simulink model "AcmotorVCO11"  (R2021a)
settings: Solver=VariableStepAuto  StartTime=0.0  StopTime=10.0  RelTol=1e-3
libraries: commsynccomp2 x3, spsAsynchronousMachinepuUnitsLib x1, spsDCVoltageSourceLib x1, spsMultimeterLib x1, pid_lib x1, spsPWMGenerator2LevelLib x1, dspstat3 x1, simulink x1, spsUniversalBridgeLib x1, spspowerguiLib x1
settings Model: Creator=User  LastModifiedBy=User

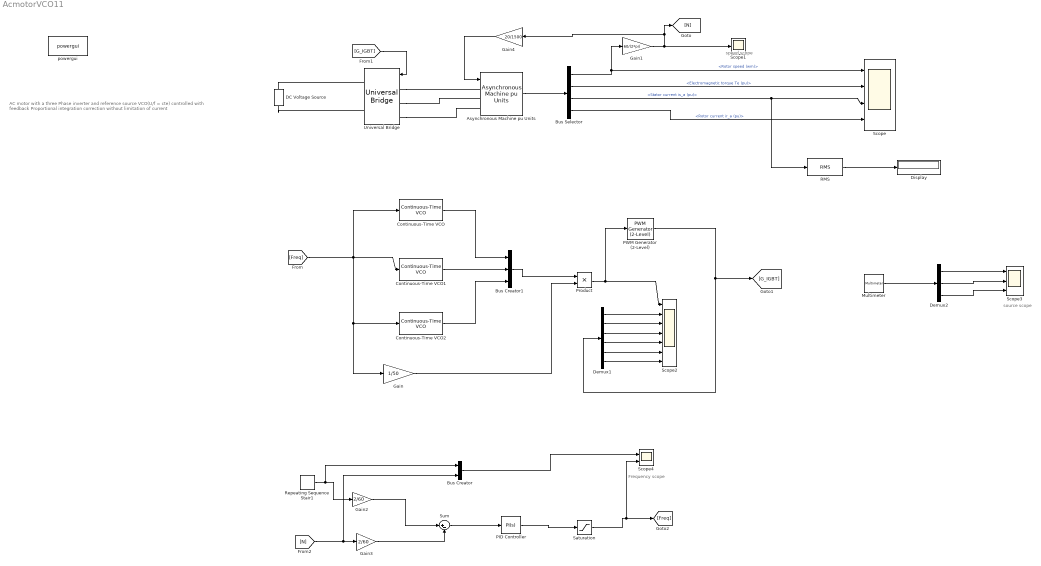
== system AcmotorVCO11 ==
  note: AC motor with a three Phase inverter and reference source VCO(U/f = cte) controlled with feedback
      | Proportional integration correction without limitation of current
  note: source scope
  note: Frequency scope
  note: speed scope
  Asynchronous Machine pu Units : spsAsynchronousMachinepuUnitsLib/Asynchronous Machine pu Units  RotorType=Squirrel-cage  PresetModel="16:  10 HP (7.5KW)  400 V 50Hz 1440 RPM"  MechanicalLoad=Torque Tm  ShowDetailedParameters=on  ReferenceFrame=Rotor  Units=pu  MeasurementBus=off  NominalParameters=[7500 400 50]  VoltageRatio=1  Stator=[0.03461 0.04484]  Rotor=[0.0347 0.04484]  Cage1=[0.01909 0.0397]  Cage2=[0.01909 0.0397]  Lm=1.827  Mechanical=[0.05642 0.001655 2]  PolePairs=2  InitialConditions="[ 1,0   0,0,0   0,0,0 ]"  SimulateSaturation=off  Saturation="[0.212,0.4201,0.8125,1.0979,1.4799,2.2457,3.2586,4.5763,6.4763 ;   0.5,0.7,0.9,1,1.1,1.2 ,1.3,1.4,1.5]"  LoadFlowParameters=0  TsPowergui=0  TsBlock=-1  IterativeModel=Trapezoidal non iterative  IterativeDiscreteModel=Trapezoidal non iterative  Pmec=0
      settings: SourceProductBaseCode=PS
  Bus Creator : BusCreator  Inputs=2
  Bus Creator1 : BusCreator  Inputs=3
  Bus Selector : BusSelector  OutputSignals=Mechanical.Rotor speed (wm),Mechanical.Electromagnetic torque Te (pu),Stator measurements.Stator current is_a (pu),Rotor measurements.Rotor current ir_a (pu)
  Continuous-Time VCO : commsynccomp2/Continuous-Time VCO  Ac=1  Fc=1  Kc=1  Ph=0
      settings: SourceProductBaseCode=CM
  Continuous-Time VCO1 : commsynccomp2/Continuous-Time VCO  Ac=1  Fc=1  Kc=1  Ph=-2*pi/3
      settings: SourceProductBaseCode=CM
  Continuous-Time VCO2 : commsynccomp2/Continuous-Time VCO  Ac=1  Fc=1  Kc=1  Ph=-4*pi/3
      settings: SourceProductBaseCode=CM
  DC Voltage Source : spsDCVoltageSourceLib/DC Voltage Source  Amplitude=600  Measurements=None
  Demux1 : Demux  Outputs=6
  Demux2 : Demux  Outputs=3
  Display : Display
  Gain : Gain  Gain=1/50
  Gain1 : Gain  Gain=60/(2*pi)
  Gain2 : Gain  Gain=2/60
  Gain3 : Gain  Gain=2/60
  Gain4 : Gain  Gain=20/1500
  Multimeter : spsMultimeterLib/Multimeter  PhasorSimulation=off  OutputType=Complex  sel=[1 2 3]  L=4  Gain=[1 1 1]  yselected={'Uab: Universal Bridge','Ubc: Universal Bridge','Uca: Universal Bridge'};  PSBOutputType=1  PSBequivalent=0  AxesSetting=[0,0.1,-100,100]  Display=0  SavedBlockNames=-11
  PID Controller : pid_lib/PID Controller  Controller=PI  Form=Parallel  TimeDomain=Continuous-time  UseExternalTs=off  SampleTime=-1  IntegratorMethod=Forward Euler  FilterMethod=Forward Euler  ControllerParametersSource=internal  P=20  I=3  D=0  UseFilter=on  N=100  TunerSelectOption=Transfer Function Based (PID Tuner App)  InitialConditionSource=internal  InitialConditionForIntegrator=0  InitialConditionForFilter=0  DifferentiatorICPrevScaledInput=0  ExternalReset=none  TrackingMode=off  Kt=1  LimitOutput=off  SatLimitsSource=internal  UpperSaturationLimit=inf  LowerSaturationLimit=-inf  LinearizeAsGain=on  AntiWindupMode=none  Kb=1  POutMin=[]  POutMax=[]  IOutMin=[]  IOutMax=[]  DOutMin=[]  DOutMax=[]  NOutMin=[]  NOutMax=[]  SumOutMin=[]  SumOutMax=[]  SaturationOutMin=[]  SaturationOutMax=[]  PParamMin=[]  PParamMax=[]  IParamMin=[]  IParamMax=[]  DParamMin=[]  DParamMax=[]  NParamMin=[]  NParamMax=[]  KbParamMin=[]  KbParamMax=[]  KtParamMin=[]  KtParamMax=[]  KbOutMin=[]  KbOutMax=[]  KtOutMin=[]  KtOutMax=[]  IntegratorOutMin=[]  IntegratorOutMax=[]  FilterOutMin=[]  FilterOutMax=[]  SumI1OutMin=[]  SumI1OutMax=[]  SumI2OutMin=[]  SumI2OutMax=[]  SumI3OutMin=[]  SumI3OutMax=[]  SumI4OutMin=[]  SumI4OutMax=[]  SumDOutMin=[]  SumDOutMax=[]  DifferentiatorOutMin=[]  DifferentiatorOutMax=[]  FilterDiffOutCoefMin=[]  FilterDiffOutCoefMax=[]  ReciprocalOutMin=[]  ReciprocalOutMax=[]  SumDenOutMin=[]  SumDenOutMax=[]  SumNumOutMin=[]  SumNumOutMax=[]  DivideOutMin=[]  DivideOutMax=[]  UdiffTsProdOutMin=[]  UdiffTsProdOutMax=[]  NTsProdOutMin=[]  NTsProdOutMax=[]  UintegralTsProdOutMin=[]  UintegralTsProdOutMax=[]  UngainTsProdOutMin=[]  UngainTsProdOutMax=[]  IntegratorContinuousStateAttributes=''  IntegratorStateMustResolveToSignalObject=off  IntegratorRTWStateStorageClass=Auto  FilterContinuousStateAttributes=''  FilterStateMustResolveToSignalObject=off  FilterRTWStateStorageClass=Auto  ParallelPVariant=InternalParameters  IdealPVariant=Disabled  IVariant=InternalParameters  DVariant=Disabled  IntegratorVariant=Continuous  SatVariant=Disabled  AWVariant=Passthrough  PCopyVariant=Disabled  TRVariant=Disabled  FdbkBlocksVariant=Forward  IdealPFdbkVariant=Disabled  SatFdbkVariant=Disabled  DerivativeFilterVariant=Disabled  NVariant=Disabled  NCopyVariant=Disabled_SignalSpec  FilterICVariant=Disabled  IntegratorICVariant=InternalICs  ExternalResetVariant=Disabled  TRSumVariant=Passthrough  SumFdbkVariant=Disabled  SumVariant=Sum_PI  TsampFilterVariant=InternalTs  TsampNgainVariant=Passthrough  TsampIntegralVariant=Passthrough  ExternalSaturationOutDataTypeStr=Inherit: Same as second input
  PWM Generator (2-Level) : spsPWMGenerator2LevelLib/PWM Generator (2-Level)  ModulatorType=Three-phase bridge (6 pulses)  ModulatorMode=Unsynchronized  Fc=1000  Pc=0  nF=27  MinMax="[ -1  1 ]"  SamplingTechnique=Natural  ModulatingSignals=off  m=0.8  Freq=60  Phase=0  Ts=0  ShowCarrierOutport=off
  Product : Product
  RMS : dspstat3/RMS  run=off  directionMode=Each column  dimension=1  InputProcessing=Columns as channels (frame based)  reset_popup=None
  Repeating Sequence Stair1 : simulink/Sources/Repeating Sequence Stair  OutValues=[1200 -1200 1200 ].'  tsamp=2  OutMin=[]  OutMax=[]  OutDataTypeStr=double  OutputDataTypeScalingMode=double  OutDataType=fixdt(0,8)  ConRadixGroup=Best Precision: Vector-wise  OutScaling=2^-12
  Saturation : Saturate  UpperLimit=60  LowerLimit=-60
  Scope : Scope  NumInputPorts=4
  Scope1 : Scope
  Scope2 : Scope  NumInputPorts=7
  Scope3 : Scope  NumInputPorts=3
  Scope4 : Scope  NumInputPorts=2
  Sum : Sum  Inputs=|+-
  Universal Bridge : spsUniversalBridgeLib/Universal Bridge  Arms=3  SnubberResistance=1e5  SnubberCapacitance=inf  Device=IGBT / Diodes  Ron=1e-3  Lon=0  ForwardVoltages="[  0  0  ]"  ForwardVoltage=0  GTOparameters=[ 10e-6 , 20e-6 ]  IGBTparameters=[ 1e-6 , 2e-6 ]  Measurements=UAB UBC UCA UDC voltages  Measurements_2=None  converterType=Rectifier
  powergui : spspowerguiLib/powergui  Priority=1  SimulationMode=Continuous  SampleTime=50e-6  frequency=60  Iterations=50  frequencyindice=50  Pbase=100e6  ErrMax=1e-4  UnitsV=kV  UnitsW=MW  buscounter=0  FunctionMessages=off  echomessages=off  EnableUseOfTLC=off  CurrentSourceSwitches=off  DisableSnubberDevices=off  DisableRonSwitches=off  DisableVfSwitches=off  DisplayEquations=off  AutomaticDiscreteSolvers=off  SolverType=Tustin/Backward Euler (TBE)  Interpol=off  ExternalGateDelay=off  methode=off  Ts=100  x0status=blocks  SPID=on  SwTol=0  HookPort=off  NonlinearTolerance=1e-4  nMaxIteration=100  ContinueOnMaxIteration=off  RestoreLinks=warning  ResistiveCurrentMeasurement=off  Frange=[0:2:500]  Ylog=off  Xlog=on  ShowGrid=off  save=off  variable=ZData  structure=0  ZoomFFT=off  StartTime=0.0  cycles=1  DisplayStyle=1  fundamental=60  FreqAxis=off  MaxFrequency=1000  frequencyindicesteady=1  RmsSteady=1  display=off
  wires:
  Continuous-Time VCO2/1 -> Bus Creator1/3
  PID Controller/1 -> Saturation/1
  Repeating Sequence Stair1/1 -> Bus Creator/1, Gain2/1
  Gain3/1 -> Sum/2
  RMS/1 -> Display/1
  Gain2/1 -> Sum/1
  Bus Creator1/1 -> Product/1
  Asynchronous Machine pu Units/1 -> Bus Selector/1
  Demux1/2 -> Scope2/3
  Demux1/4 -> Scope2/5
  Continuous-Time VCO1/1 -> Bus Creator1/2
  Continuous-Time VCO/1 -> Bus Creator1/1
  Bus Selector/2 -> Scope/2  "<Electromagnetic torque Te (pu)>"
  Demux1/1 -> Scope2/2
  [N] -> Bus Creator/2, Gain3/1
  Demux1/6 -> Scope2/7
  Bus Creator/1 -> Scope4/1
  Bus Selector/1 -> Gain1/1, Scope/1  "<Rotor speed (wm)>"
  PWM Generator (2-Level)/1 -> Demux1/1, [G_IGBT]
  Demux1/3 -> Scope2/4
  Saturation/1 -> Scope4/2, [Freq]
  Demux2/3 -> Scope3/3
  Bus Selector/4 -> Scope/4  "<Rotor current ir_a (pu)>"
  Sum/1 -> PID Controller/1
  Product/1 -> PWM Generator (2-Level)/1, Scope2/1
  Demux1/5 -> Scope2/6
  [G_IGBT] -> Universal Bridge/1
  Gain/1 -> Product/2
  Gain1/1 -> [N], Gain4/1, Scope1/1
  [Freq] -> Gain/1, Continuous-Time VCO2/1, Continuous-Time VCO1/1, Continuous-Time VCO/1
  Multimeter/1 -> Demux2/1
  Demux2/2 -> Scope3/2
  Bus Selector/3 -> RMS/1, Scope/3  "<Stator current is_a (pu)>"
  Demux2/1 -> Scope3/1
  Gain4/1 -> Asynchronous Machine pu Units/1
  connections:
  Universal Bridge/LConn2 -- Asynchronous Machine pu Units/LConn2
  Universal Bridge/LConn1 -- Asynchronous Machine pu Units/LConn1
  DC Voltage Source/RConn1 -- Universal Bridge/RConn1
  Universal Bridge/LConn3 -- Asynchronous Machine pu Units/LConn3
  DC Voltage Source/LConn1 -- Universal Bridge/RConn2
